simulink model "q7_compare"  (R2021a)
settings: Solver=VariableStepAuto  StartTime=0.0  StopTime=30  RelTol=1e-3
libraries: cstblocks x5, pid_lib x1
settings Model: Creator=mj_sh  LastModifiedBy=mj_sh

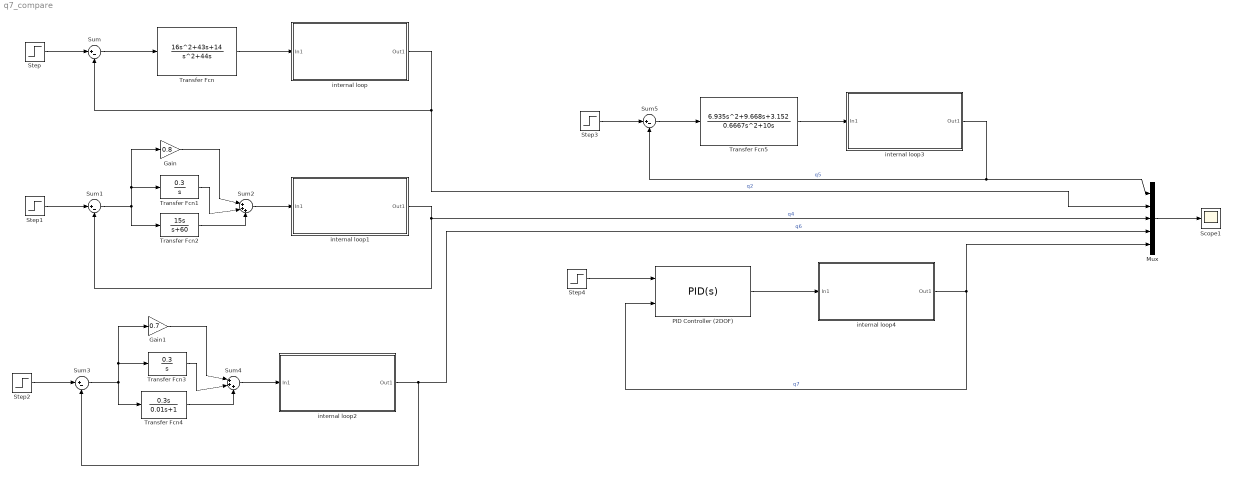
== system q7_compare ==
  Gain : Gain  Gain=0.8
  Gain1 : Gain  Gain=0.7
  Mux : Mux  Inputs=5
  PID Controller (2DOF) : pid_lib/PID Controller (2DOF)  Controller=PID  Form=Parallel  TimeDomain=Continuous-time  UseExternalTs=off  SampleTime=-1  IntegratorMethod=Forward Euler  FilterMethod=Forward Euler  ControllerParametersSource=internal  P=1.91206426119348  I=0.218784094899679  D=4.04275038096098  UseFilter=on  N=121.379989923856  b=1.20927644511706  c=0.0366462486007094  TunerSelectOption=Transfer Function Based (PID Tuner App)  InitialConditionSource=internal  InitialConditionForIntegrator=0  InitialConditionForFilter=0  DifferentiatorICPrevScaledInput=0  ExternalReset=none  TrackingMode=off  Kt=1  LimitOutput=off  SatLimitsSource=internal  UpperSaturationLimit=inf  LowerSaturationLimit=-inf  LinearizeAsGain=on  AntiWindupMode=none  Kb=1  POutMin=[]  POutMax=[]  IOutMin=[]  IOutMax=[]  DOutMin=[]  DOutMax=[]  NOutMin=[]  NOutMax=[]  bOutMin=[]  bOutMax=[]  cOutMin=[]  cOutMax=[]  SumOutMin=[]  SumOutMax=[]  SaturationOutMin=[]  SaturationOutMax=[]  PParamMin=[]  PParamMax=[]  IParamMin=[]  IParamMax=[]  DParamMin=[]  DParamMax=[]  NParamMin=[]  NParamMax=[]  bParamMin=[]  bParamMax=[]  cParamMin=[]  cParamMax=[]  KbParamMin=[]  KbParamMax=[]  KtParamMin=[]  KtParamMax=[]  KbOutMin=[]  KbOutMax=[]  KtOutMin=[]  KtOutMax=[]  IntegratorOutMin=[]  IntegratorOutMax=[]  FilterOutMin=[]  FilterOutMax=[]  SumI1OutMin=[]  SumI1OutMax=[]  SumI2OutMin=[]  SumI2OutMax=[]  SumI3OutMin=[]  SumI3OutMax=[]  SumI4OutMin=[]  SumI4OutMax=[]  SumDOutMin=[]  SumDOutMax=[]  Sum1OutMin=[]  Sum1OutMax=[]  Sum2OutMin=[]  Sum2OutMax=[]  Sum3OutMin=[]  Sum3OutMax=[]  DifferentiatorOutMin=[]  DifferentiatorOutMax=[]  FilterDiffOutCoefMin=[]  FilterDiffOutCoefMax=[]  ReciprocalOutMin=[]  ReciprocalOutMax=[]  SumDenOutMin=[]  SumDenOutMax=[]  SumNumOutMin=[]  SumNumOutMax=[]  DivideOutMin=[]  DivideOutMax=[]  UdiffTsProdOutMin=[]  UdiffTsProdOutMax=[]  NTsProdOutMin=[]  NTsProdOutMax=[]  UintegralTsProdOutMin=[]  UintegralTsProdOutMax=[]  UngainTsProdOutMin=[]  UngainTsProdOutMax=[]  IntegratorContinuousStateAttributes=''  IntegratorStateMustResolveToSignalObject=off  IntegratorRTWStateStorageClass=Auto  FilterContinuousStateAttributes=''  FilterStateMustResolveToSignalObject=off  FilterRTWStateStorageClass=Auto  ParallelPVariant=InternalParameters  IdealPVariant=Disabled  IVariant=InternalParameters  DVariant=InternalParameters  bVariant=InternalParameters  cVariant=InternalParameters  IntegratorVariant=Continuous  SatVariant=Disabled  AWVariant=Passthrough  PCopyVariant=Disabled  TRVariant=Disabled  FdbkBlocksVariant=Forward  IdealPFdbkVariant=Disabled  SatFdbkVariant=Disabled  DerivativeFilterVariant=ContFilter  NVariant=InternalParameters  NCopyVariant=Disabled  FilterICVariant=InternalICsFilter  IntegratorICVariant=InternalICs  ExternalResetVariant=Disabled  TRSumVariant=Passthrough  SumFdbkVariant=Disabled  SumVariant=Sum_PID  TsampFilterVariant=InternalTs  TsampNgainVariant=Passthrough  TsampIntegralVariant=Passthrough  ExternalSaturationOutDataTypeStr=Inherit: Same as second input
      settings: SourceProductBaseCode=SL
  Scope1 : Scope
  Step{,1..4} (5 alike) : Step  Time=0  After=0.5  SampleTime=0
  Sum{,1,3,5} (4 alike) : Sum  Inputs=|+-
  Sum2 : Sum  Inputs=|+++
  Sum4 : Sum  Inputs=|+++
  Transfer Fcn : TransferFcn  Numerator=[16 43 14]  Denominator=[1 44 0]
  Transfer Fcn1 : TransferFcn  Numerator=[0.3]  Denominator=[1 0]
  Transfer Fcn2 : TransferFcn  Numerator=[15 0]  Denominator=[1 60]
  Transfer Fcn3 : TransferFcn  Numerator=[0.3]  Denominator=[1 0]
  Transfer Fcn4 : TransferFcn  Numerator=[0.3 0]  Denominator=[0.01 1]
  Transfer Fcn5 : TransferFcn  Numerator=[6.935 9.668 3.152]  Denominator=[0.6667 10 0]
  internal loop : Subsystem
  internal loop1 : Subsystem
  internal loop2 : Subsystem
  internal loop3 : Subsystem
  internal loop4 : Subsystem
  wires:
  Step/1 -> Sum/1
  Sum/1 -> Transfer Fcn/1
  Transfer Fcn/1 -> internal loop/1(In1)
  internal loop/1(Out1) -> Mux/2, Sum/2  "q2"
  internal loop1/1(Out1) -> Mux/3, Sum1/2  "q4"
  Step1/1 -> Sum1/1
  Sum1/1 -> Transfer Fcn2/1, Transfer Fcn1/1, Gain/1
  Sum2/1 -> internal loop1/1(In1)
  Gain/1 -> Sum2/1
  Transfer Fcn1/1 -> Sum2/2
  Transfer Fcn2/1 -> Sum2/3
  Transfer Fcn4/1 -> Sum4/3
  Transfer Fcn3/1 -> Sum4/2
  Gain1/1 -> Sum4/1
  Sum4/1 -> internal loop2/1(In1)
  Sum3/1 -> Gain1/1, Transfer Fcn3/1, Transfer Fcn4/1
  Step2/1 -> Sum3/1
  internal loop2/1(Out1) -> Mux/4, Sum3/2  "q6"
  internal loop3/1(Out1) -> Mux/1, Sum5/2  "q5"
  Transfer Fcn5/1 -> internal loop3/1(In1)
  Sum5/1 -> Transfer Fcn5/1
  Step3/1 -> Sum5/1
  PID Controller (2DOF)/1 -> internal loop4/1(In1)
  internal loop4/1(Out1) -> Mux/5, PID Controller (2DOF)/2  "q7"
  Step4/1 -> PID Controller (2DOF)/1
  Mux/1 -> Scope1/1

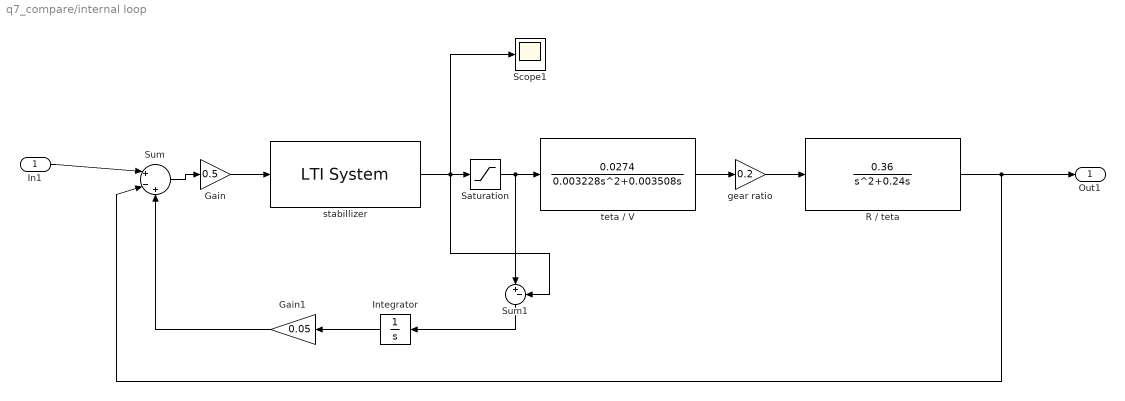
== system q7_compare/internal loop ==
  In1 : Inport
  Gain : Gain  Gain=0.5
  Gain1 : Gain  Gain=0.05
  Integrator : Integrator
  R / teta : TransferFcn  Numerator=[0.36]  Denominator=[1 0.24 0]
  Saturation : Saturate  UpperLimit=20  LowerLimit=-20
  Scope1 : Scope
  Sum : Sum  Inputs=|+-+
  Sum1 : Sum  Inputs=|+-
  gear ratio : Gain  Gain=0.2
  stabillizer : cstblocks/LTI System  sys=K  IC=[]
  teta / V : TransferFcn  Numerator=[0.0274]  Denominator=[0.003228 0.003508 0]
  Out1 : Outport
  wires:
  Gain/1 -> stabillizer/1
  Saturation/1 -> teta / V/1, Sum1/1
  Integrator/1 -> Gain1/1
  Sum1/1 -> Integrator/1
  gear ratio/1 -> R / teta/1
  stabillizer/1 -> Scope1/1, Sum1/2, Saturation/1
  Sum/1 -> Gain/1
  R / teta/1 -> Out1/1, Sum/2
  Gain1/1 -> Sum/3
  teta / V/1 -> gear ratio/1
  In1/1 -> Sum/1

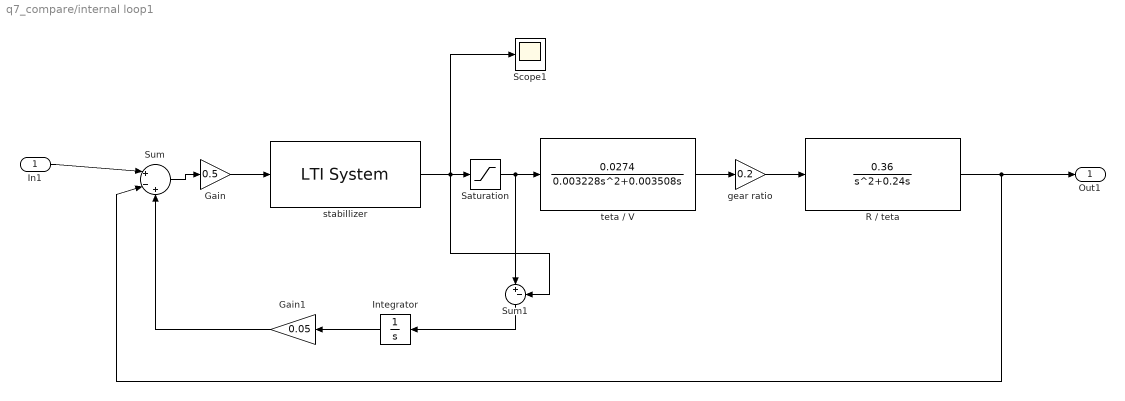
== system q7_compare/internal loop1 ==
  In1 : Inport
  Gain : Gain  Gain=0.5
  Gain1 : Gain  Gain=0.05
  Integrator : Integrator
  R / teta : TransferFcn  Numerator=[0.36]  Denominator=[1 0.24 0]
  Saturation : Saturate  UpperLimit=20  LowerLimit=-20
  Scope1 : Scope
  Sum : Sum  Inputs=|+-+
  Sum1 : Sum  Inputs=|+-
  gear ratio : Gain  Gain=0.2
  stabillizer : cstblocks/LTI System  sys=K  IC=[]
  teta / V : TransferFcn  Numerator=[0.0274]  Denominator=[0.003228 0.003508 0]
  Out1 : Outport
  wires:
  In1/1 -> Sum/1
  teta / V/1 -> gear ratio/1
  Gain1/1 -> Sum/3
  R / teta/1 -> Sum/2, Out1/1
  Sum/1 -> Gain/1
  stabillizer/1 -> Saturation/1, Sum1/2, Scope1/1
  gear ratio/1 -> R / teta/1
  Sum1/1 -> Integrator/1
  Integrator/1 -> Gain1/1
  Saturation/1 -> Sum1/1, teta / V/1
  Gain/1 -> stabillizer/1

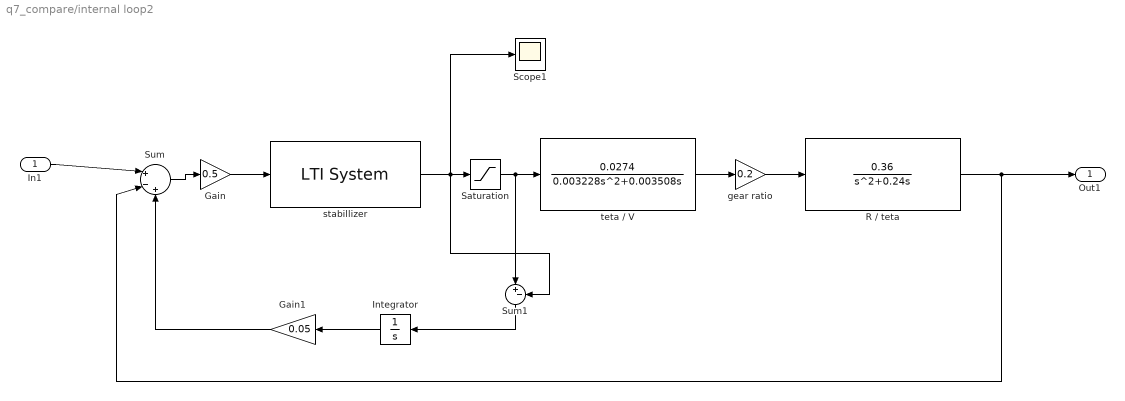
== system q7_compare/internal loop2 ==
  In1 : Inport
  Gain : Gain  Gain=0.5
  Gain1 : Gain  Gain=0.05
  Integrator : Integrator
  R / teta : TransferFcn  Numerator=[0.36]  Denominator=[1 0.24 0]
  Saturation : Saturate  UpperLimit=20  LowerLimit=-20
  Scope1 : Scope
  Sum : Sum  Inputs=|+-+
  Sum1 : Sum  Inputs=|+-
  gear ratio : Gain  Gain=0.2
  stabillizer : cstblocks/LTI System  sys=K  IC=[]
  teta / V : TransferFcn  Numerator=[0.0274]  Denominator=[0.003228 0.003508 0]
  Out1 : Outport
  wires:
  Gain/1 -> stabillizer/1
  Saturation/1 -> teta / V/1, Sum1/1
  Integrator/1 -> Gain1/1
  Sum1/1 -> Integrator/1
  gear ratio/1 -> R / teta/1
  stabillizer/1 -> Scope1/1, Sum1/2, Saturation/1
  Sum/1 -> Gain/1
  R / teta/1 -> Out1/1, Sum/2
  Gain1/1 -> Sum/3
  teta / V/1 -> gear ratio/1
  In1/1 -> Sum/1

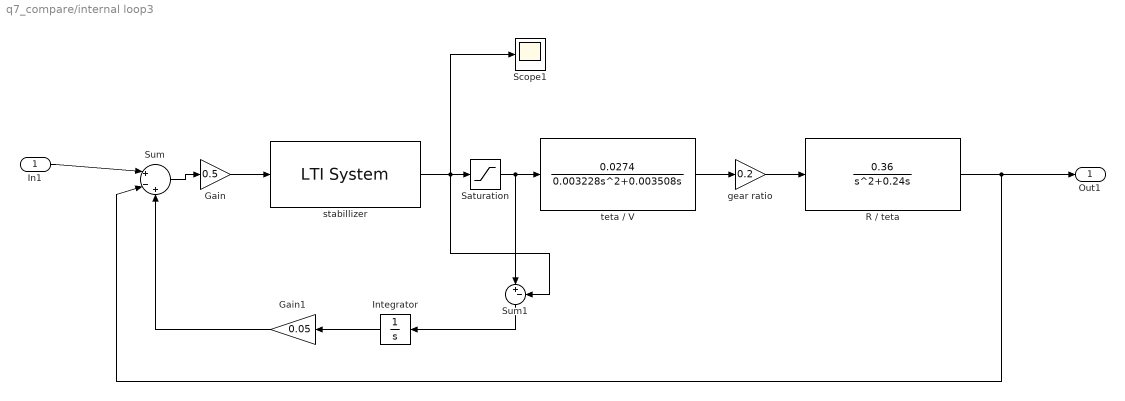
== system q7_compare/internal loop3 ==
  In1 : Inport
  Gain : Gain  Gain=0.5
  Gain1 : Gain  Gain=0.05
  Integrator : Integrator
  R / teta : TransferFcn  Numerator=[0.36]  Denominator=[1 0.24 0]
  Saturation : Saturate  UpperLimit=20  LowerLimit=-20
  Scope1 : Scope
  Sum : Sum  Inputs=|+-+
  Sum1 : Sum  Inputs=|+-
  gear ratio : Gain  Gain=0.2
  stabillizer : cstblocks/LTI System  sys=K  IC=[]
  teta / V : TransferFcn  Numerator=[0.0274]  Denominator=[0.003228 0.003508 0]
  Out1 : Outport
  wires:
  In1/1 -> Sum/1
  teta / V/1 -> gear ratio/1
  Gain1/1 -> Sum/3
  R / teta/1 -> Sum/2, Out1/1
  Sum/1 -> Gain/1
  stabillizer/1 -> Saturation/1, Sum1/2, Scope1/1
  gear ratio/1 -> R / teta/1
  Sum1/1 -> Integrator/1
  Integrator/1 -> Gain1/1
  Saturation/1 -> Sum1/1, teta / V/1
  Gain/1 -> stabillizer/1

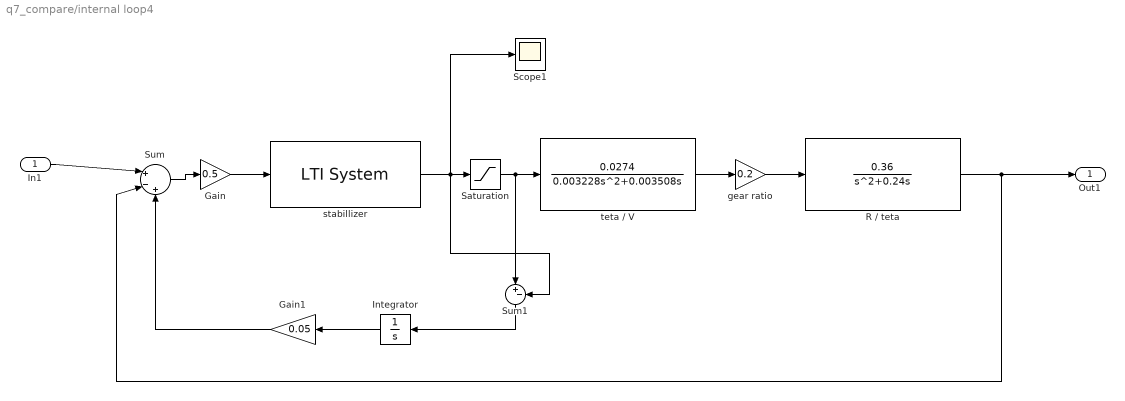
== system q7_compare/internal loop4 ==
  In1 : Inport
  Gain : Gain  Gain=0.5
  Gain1 : Gain  Gain=0.05
  Integrator : Integrator
  R / teta : TransferFcn  Numerator=[0.36]  Denominator=[1 0.24 0]
  Saturation : Saturate  UpperLimit=20  LowerLimit=-20
  Scope1 : Scope
  Sum : Sum  Inputs=|+-+
  Sum1 : Sum  Inputs=|+-
  gear ratio : Gain  Gain=0.2
  stabillizer : cstblocks/LTI System  sys=K  IC=[]
  teta / V : TransferFcn  Numerator=[0.0274]  Denominator=[0.003228 0.003508 0]
  Out1 : Outport
  wires:
  Gain/1 -> stabillizer/1
  Saturation/1 -> teta / V/1, Sum1/1
  Integrator/1 -> Gain1/1
  Sum1/1 -> Integrator/1
  gear ratio/1 -> R / teta/1
  stabillizer/1 -> Scope1/1, Sum1/2, Saturation/1
  Sum/1 -> Gain/1
  R / teta/1 -> Out1/1, Sum/2
  Gain1/1 -> Sum/3
  teta / V/1 -> gear ratio/1
  In1/1 -> Sum/1
